simulink model "Edited_MotorXploer"  (R2024b)
settings: Solver=FixedStepAuto  StartTime=0.0  StopTime=10  FixedStep=0.001  RelTol=1e-3
undefined symbols (not defined in the file or in its folder): Blocking, LF, Non
libraries: hdlsllib x5, amg_usbconverter_n_connect_lib x3, dspfdesign x1
settings Model: Creator=beamk  LastModifiedBy=charmil

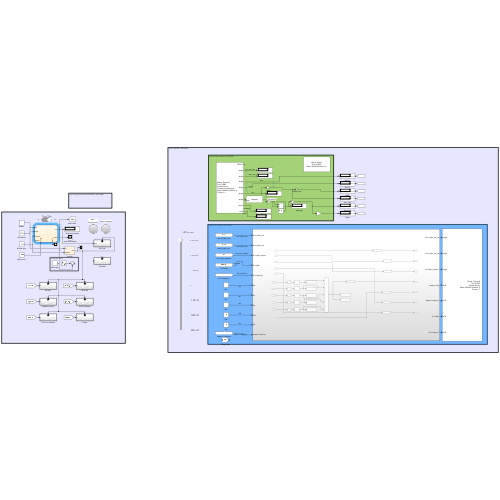
[thumbnail: Simulink's stored preview of the top-level diagram]
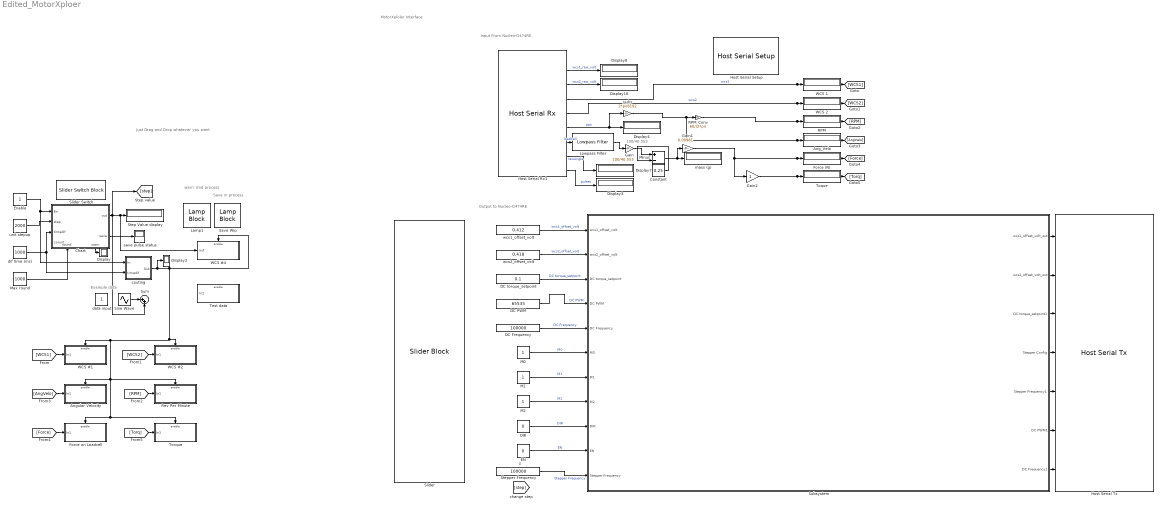
== system Edited_MotorXploer ==
  note: 0
  note: 100/40.553
  note: Just Drag and Drop whatever you want
  note: Output to Nucleo-G474RE
  note: Input From Nucleo-G474RE
  note: MotorXploler Interface
  note: Save in process
  note: Example data
  note: warn:
      | End process
  Ang_Velo : Display
  Angular Velocity : Subsystem  TreatAsAtomicUnit=on
  Chart : Stateflow chart  TreatAsAtomicUnit=on
      settings: PortSchema="{\"entries\":[{\"content\":{\"sides\":[{\"content\":{\"connectorIds\":[\"In2\",\"In3\",\"In4\",\"In5\"]},\"type\":\"ConnectorPlacement.EquallySpacedRectSide\",\"uuid\":\"dac77e3e-29fa-48b2-8dbc-87de7162ff91\"},{\"content\":{\"connectorIds\":[\"Out3\",\"Out2\"],\"side\":\"RIGHT\"},\"type\":\"ConnectorPlacement.EquallySpacedRectSide\",\"uuid\":\"95dcbdb3-8d7f-4284-beec-a5517aef8ac9\"},{\"content\":{\"side\":\"TOP\"},\"type\":\"ConnectorPlacement.EquallySpacedRectSide\",\"uuid\":\"16d4b6a6-1864-4ff8-80c4-a30afaa9113f\"},{\"content\":{\"connectorIds\":[\"In1\",\"Out1\"],\"side\":\"BOTTOM\"},\"type\":\"ConnectorPlacement.EquallySpacedRectSide\",\"uuid\":\"ee49f440-8a25-4cdc-af3c-34657fa2d15f\"}]},\"type\":\"ConnectorPlacement.EquallySpacedConnector\",\"uuid\":\"13973787-06fa-47f1-9425-9f6e417a8e61\"}],\"packageUris\":[\"http://schema.mathworks.com/mf0/Connector/R2020b\"],\"version\":\"1.0\"}"
  Constant : Constant  Value=0.25
  DC Frequency : Constant  Value=100000
  DC PWM : Constant  Value=65535
  DC torque_setpoint : Constant  Value=0.1
  DIR : Constant  Value=0  OutDataTypeStr=uint8
  Display{,2..4,7..8,16} (7 alike) : Display
  EN : Constant  Value=0  OutDataTypeStr=uint8
  Enable : Constant
  Force (N) : Display
  Force on Loadcell : Subsystem  TreatAsAtomicUnit=on
  Gain : Gain  Gain=100/40.553
  Gain1 : Gain  Gain=0.00981
  Gain2 : Gain
  Host Serial Rx1 : amg_usbconverter_n_connect_lib/Host Serial Rx  conf=rx  port=<auto>  baudrate=2000000  databits=8  parity=None  stopbit=1  flowcontrol=None  transfer=Non-Blocking  timeout=5  packetmode=Binary  enableinitialvalues=off  initialvalues=[]  binheader='45'  binterminator='A'  porttype_double=0  porttype_single=6  porttype_int8=0  porttype_uint8=0  porttype_int16=0  porttype_uint16=1  porttype_int32=1  porttype_uint32=0  asciiformat='%f,%f,%d,%d'  rx_asciiterminator="LF (0x0A - \"\\n\")"  tx_asciiterminator="CRLF (0x0D 0x0A - \"\\r\\n\")"  sampletime=-1  enablecustomportlabel=off  cinputportlabel=0  coutputportlabel=A  portpinstr=0  blockid=HostSerialRx1  inputporttype=[]  inputportwidth=[]  inputportlabel={}  outputporttype=[3 1 1 1 1 1 1 5 6]  outputportwidth=[1 1 1 1 1 1 1 1 1]  outputportlabel={'READY','single','single','single','single','single','single','uint16','int32'}  compat=0  optionstring=[]  autoport='COM3'
  Host Serial Setup : amg_usbconverter_n_connect_lib/Host Serial Setup  conf=setup  port=<auto>  baudrate=2000000  databits=8  parity=None  stopbit=1  flowcontrol=None  transfer=Blocking  timeout=2  packetmode=Binary  initialvalues=[]  binheader='7E 7E'  binterminator='03 03'  porttype_double=0  porttype_single=1  porttype_int8=0  porttype_uint8=0  porttype_int16=0  porttype_uint16=0  porttype_int32=0  porttype_uint32=2  asciiformat='%d %u %x'  rx_asciiterminator="CRLF (0x0D 0x0A - \"\\r\\n\")"  tx_asciiterminator="CRLF (0x0D 0x0A - \"\\r\\n\")"  sampletime=-1  enablecustomportlabel=off  cinputportlabel=0  coutputportlabel=A  portpinstr=0  blockid=HostSerialSetup  inputporttype=[]  inputportwidth=[]  inputportlabel={}  outputporttype=[]  outputportwidth=[]  outputportlabel={}  compat=0  optionstring=[]  autoport='COM3'
  Host Serial Tx : amg_usbconverter_n_connect_lib/Host Serial Tx  conf=tx  port=<auto>  baudrate=2000000  databits=8  parity=None  stopbit=1  flowcontrol=None  transfer=Blocking  timeout=2  packetmode=Binary  initialvalues=[]  binheader='45'  binterminator='A'  porttype_double=0  porttype_single=3  porttype_int8=0  porttype_uint8=1  porttype_int16=0  porttype_uint16=0  porttype_int32=3  porttype_uint32=0  asciiformat='%d,%f'  rx_asciiterminator="CRLF (0x0D 0x0A - \"\\r\\n\")"  tx_asciiterminator="CRLF (0x0D 0x0A - \"\\r\\n\")"  sampletime=-1  enablecustomportlabel=off  cinputportlabel=0  coutputportlabel=A  portpinstr=0  blockid=HostSerialTx  inputporttype=[1 1 1 3 6 6 6]  inputportwidth=[1 1 1 1 1 1 1]  inputportlabel={'single','single','single','uint8','int32','int32','int32'}  outputporttype=[]  outputportwidth=[]  outputportlabel={}  compat=0  optionstring=[]  autoport='COM3'
      settings: SourceProductName=aMG USB Converter N
  Lamp1 : LampBlock  LabelPosition=Hide
  Lowpass Filter : dspfdesign/Lowpass Filter  FilterType=FIR  DesignForMinimumOrder=on  FilterOrder=50  PassbandFrequency=0.01  StopbandFrequency=0.1  PassbandRipple=0.1  StopbandAttenuation=80  SampleRateMode=Use normalized frequency (0 to 1)  SampleRate=44100  SimulateUsing=Interpreted execution  roundingMode=Floor  coeffsDataTypeStr=fixdt(1,16)
  M0 : Constant  OutDataTypeStr=uint8
  M1 : Constant
  M2 : Constant  OutDataTypeStr=uint8
  Max round : Constant  Value=1000
  Minus : Sum  Inputs=+-
  RPM : Display
  RPM_Conv : Gain  Gain=60/(2*pi)
  Rev Per Minute : Subsystem  TreatAsAtomicUnit=on
  Save Wip : LampBlock  LabelPosition=Hide
  Sine Wave : Sin  Frequency=20  SampleTime=0
  Slider : SliderBlock  ScaleMin=-65535  ScaleMax=65535
  Slider Switch : SliderSwitchBlock
      settings: Values={{'Off', 'On'}, [0 1]}
  Step Value display : Display
  Stepper Frequency : Constant  Value=100000  VectorParams1D=off
  Subsystem : Subsystem
  Sum : Sum  Inputs=|++
  Test data : Subsystem  TreatAsAtomicUnit=on
  Toque : Display
  Torque : Subsystem  TreatAsAtomicUnit=on
  WCS #1 : Subsystem  TreatAsAtomicUnit=on
  WCS #2 : Subsystem  TreatAsAtomicUnit=on
  WCS #4 : Subsystem  TreatAsAtomicUnit=on
  WCS 1 : Display
  WCS 2 : Display
  couting : Stateflow chart  TreatAsAtomicUnit=on
  data input : Constant
  dif time (ms) : Constant  Value=1000
  mass (g) : Display
  rad/s : Gain  Gain=2*pi/8192
  save pulse status : Display
  unit stepup : Constant  Value=2000
  wcs1_offset_volt : Constant  Value=0.412  OutDataTypeStr=single
  wcs2_offset_volt : Constant  Value=0.418  OutDataTypeStr=single
  wires:
  Host Serial Rx1/2 -> Display8/1  "wcs1_raw_volt"
  Host Serial Rx1/3 -> Display16/1  "wcs2_raw_volt"
  Host Serial Rx1/7 -> Lowpass Filter/1  "loadcell"
  Host Serial Rx1/5 -> [WCS2], WCS 2/1  "wcs2"
  Host Serial Rx1/8 -> Display7/1  "rawAngle"
  rad/s/1 -> [AngVelo], Ang_Velo/1, RPM_Conv/1
  Host Serial Rx1/6 -> Display4/1, rad/s/1  "pps"
  Host Serial Rx1/4 -> [WCS1], WCS 1/1  "wcs1"
  Host Serial Rx1/9 -> Display3/1  "pulses"
  wcs1_offset_volt/1 -> Subsystem/1(wcs1_offset_volt)  "wcs1_offset_volt"
  wcs2_offset_volt/1 -> Subsystem/2(wcs2_offset_volt)  "wcs2_offset_volt"
  DC torque_setpoint/1 -> Subsystem/3(DC torque_setpoint)  "DC torque_setpoint"
  DC PWM/1 -> Subsystem/4(DC PWM)  "DC PWM"
  DC Frequency/1 -> Subsystem/5(DC Frequency)  "DC Frequency"
  M0/1 -> Subsystem/6(M0)  "M0"
  M1/1 -> Subsystem/7(M1)  "M1"
  M2/1 -> Subsystem/8(M2)  "M2"
  DIR/1 -> Subsystem/9(DIR)  "DIR"
  EN/1 -> Subsystem/10(EN)  "EN"
  Subsystem/1(wcs1_offset_volt_out) -> Host Serial Tx/1
  Subsystem/2(wcs2_offset_volt_out) -> Host Serial Tx/2
  Subsystem/3(DC torque_setpoint1) -> Host Serial Tx/3
  Subsystem/4(Stepper Config) -> Host Serial Tx/4
  Subsystem/5(Stepper Frequency1) -> Host Serial Tx/5
  Subsystem/6(DC PWM1) -> Host Serial Tx/6
  Subsystem/7(DC Frequency1) -> Host Serial Tx/7
  Gain/1 -> Minus/1
  Gain1/1 -> Gain2/1, [Force], Force (N)/1
  RPM_Conv/1 -> [RPM], RPM/1
  Sine Wave/1 -> Sum/1
  Chart/2(save) -> save pulse status/1
  dif time (ms)/1 -> couting/2(timedif), Chart/4(timedif)
  Chart/3(out) -> Sum/2, WCS #4/1(out), Step Value display/1, [step]
  Enable/1 -> Chart/2(En), couting/1(In)
  unit stepup/1 -> Chart/3(step)
  Gain2/1 -> [Torq], Toque/1
  [WCS1] -> WCS #1/1(In1)
  [WCS2] -> WCS #2/1(In1)
  [RPM] -> Rev Per Minute/1(In1)
  [Force] -> Force on Loadcell/1(In1)
  [Torq] -> Torque/1(In1)
  Max round/1 -> Chart/1(round)
  Chart/1(warn) -> Display/1
  Lowpass Filter/1 -> Gain/1
  Constant/1 -> Minus/2
  Minus/1 -> Gain1/1, mass (g)/1
  [AngVelo] -> Angular Velocity/1(In1)
  couting/1(Out) -> WCS #4/Enable, WCS #2/Enable, WCS #1/Enable, Angular Velocity/Enable, Rev Per Minute/Enable, Torque/Enable, Force on Loadcell/Enable, Display2/1
  Stepper Frequency/1 -> Subsystem/11(Stepper Frequency)  "Stepper Frequency"

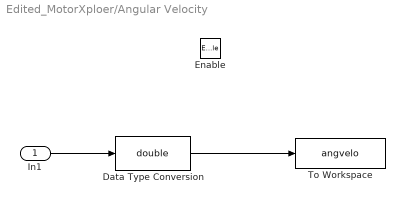
== system Edited_MotorXploer/Angular Velocity ==
  In1 : Inport
  Enable : EnablePort
  Data Type Conversion : DataTypeConversion  OutDataTypeStr=double  SaturateOnIntegerOverflow=off  RndMeth=Floor
  To Workspace : ToWorkspace  VariableName=angvelo  SampleTime=-1
      settings: Save2DSignal=2-D array (concatenate along first dimension)
  wires:
  In1/1 -> Data Type Conversion/1
  Data Type Conversion/1 -> To Workspace/1

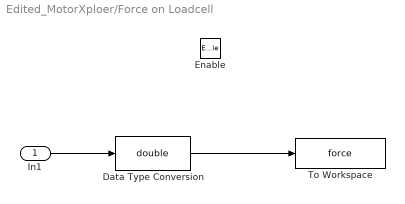
== system Edited_MotorXploer/Force on Loadcell ==
  In1 : Inport
  Enable : EnablePort
  Data Type Conversion : DataTypeConversion  OutDataTypeStr=double  SaturateOnIntegerOverflow=off  RndMeth=Floor
  To Workspace : ToWorkspace  VariableName=force  SampleTime=-1
      settings: Save2DSignal=2-D array (concatenate along first dimension)
  wires:
  In1/1 -> Data Type Conversion/1
  Data Type Conversion/1 -> To Workspace/1

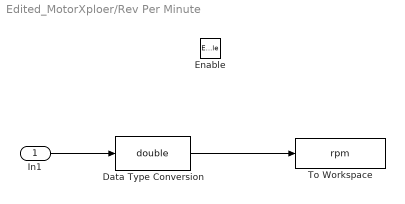
== system Edited_MotorXploer/Rev Per Minute ==
  In1 : Inport
  Enable : EnablePort
  Data Type Conversion : DataTypeConversion  OutDataTypeStr=double  SaturateOnIntegerOverflow=off  RndMeth=Floor
  To Workspace : ToWorkspace  VariableName=rpm  SampleTime=-1
      settings: Save2DSignal=2-D array (concatenate along first dimension)
  wires:
  In1/1 -> Data Type Conversion/1
  Data Type Conversion/1 -> To Workspace/1

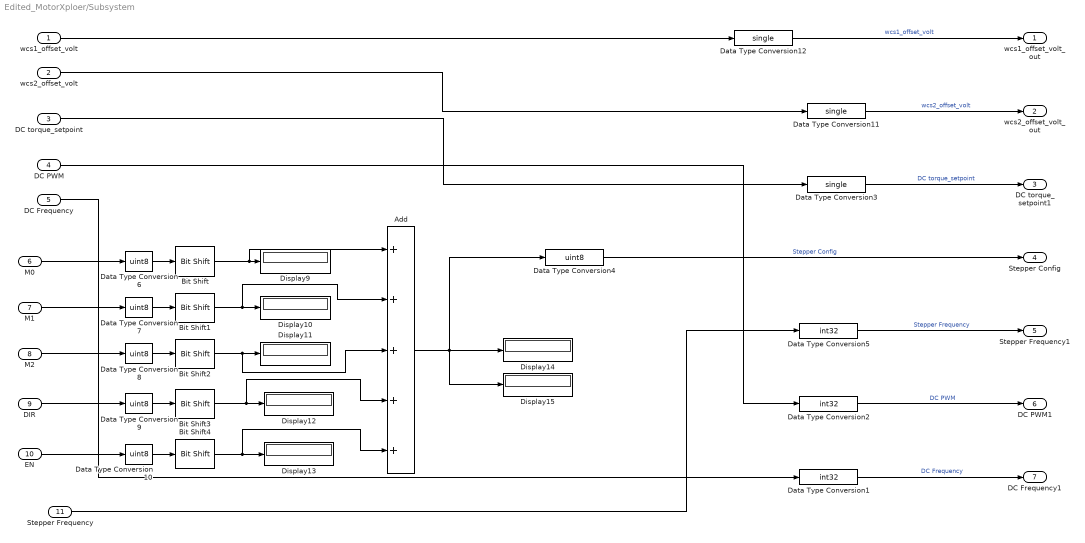
== system Edited_MotorXploer/Subsystem ==
  wcs1_offset_volt : Inport
  wcs2_offset_volt : Inport  Port=2
  DC torque_setpoint : Inport  Port=3
  DC PWM : Inport  Port=4
  DC Frequency : Inport  Port=5
  M0 : Inport  Port=6
  M1 : Inport  Port=7
  M2 : Inport  Port=8
  DIR : Inport  Port=9
  EN : Inport  Port=10
  Stepper Frequency : Inport  Port=11
  Add : Sum  Inputs=+++++
  Bit Shift : hdlsllib/Logic and Bit Operations/Bit Shift  mode=Shift Left Logical  N=4
  Bit Shift1 : hdlsllib/Logic and Bit Operations/Bit Shift  mode=Shift Left Logical  N=3
  Bit Shift2 : hdlsllib/Logic and Bit Operations/Bit Shift  mode=Shift Left Logical  N=2
  Bit Shift3 : hdlsllib/Logic and Bit Operations/Bit Shift  mode=Shift Left Logical  N=1
  Bit Shift4 : hdlsllib/Logic and Bit Operations/Bit Shift  mode=Shift Left Logical  N=0
  Data Type Conversion1 : DataTypeConversion  OutDataTypeStr=int32  SaturateOnIntegerOverflow=off  RndMeth=Floor
  Data Type Conversion{4,6..10} (6 alike) : DataTypeConversion  OutDataTypeStr=uint8  SaturateOnIntegerOverflow=off  RndMeth=Floor
  Data Type Conversion11 : DataTypeConversion  OutDataTypeStr=single  SaturateOnIntegerOverflow=off  RndMeth=Floor
  Data Type Conversion12 : DataTypeConversion  OutDataTypeStr=single  SaturateOnIntegerOverflow=off  RndMeth=Floor
  Data Type Conversion2 : DataTypeConversion  OutDataTypeStr=int32  SaturateOnIntegerOverflow=off  RndMeth=Floor
  Data Type Conversion3 : DataTypeConversion  OutDataTypeStr=single  SaturateOnIntegerOverflow=off  RndMeth=Floor
  Data Type Conversion5 : DataTypeConversion  OutDataTypeStr=int32  SaturateOnIntegerOverflow=off  RndMeth=Floor
  Display{9..15} (7 alike) : Display
      Display10 settings: Format=binary (Stored Integer)
      Display11 settings: Format=binary (Stored Integer)
      Display12 settings: Format=binary (Stored Integer)
      Display13 settings: Format=binary (Stored Integer)
      Display14 settings: Format=binary (Stored Integer)
      Display9 settings: Format=binary (Stored Integer)
  wcs1_offset_volt_out : Outport
  wcs2_offset_volt_out : Outport  Port=2
  DC torque_setpoint1 : Outport  Port=3
  Stepper Config : Outport  Port=4
  Stepper Frequency1 : Outport  Port=5
  DC PWM1 : Outport  Port=6
  DC Frequency1 : Outport  Port=7
  wires:
  Bit Shift/1 -> Display9/1, Add/1
  Data Type Conversion8/1 -> Bit Shift2/1
  EN/1 -> Data Type Conversion10/1
  Data Type Conversion6/1 -> Bit Shift/1
  DC torque_setpoint/1 -> Data Type Conversion3/1
  Data Type Conversion2/1 -> DC PWM1/1  "DC PWM"
  Data Type Conversion7/1 -> Bit Shift1/1
  Data Type Conversion10/1 -> Bit Shift4/1
  DC PWM/1 -> Data Type Conversion2/1
  Bit Shift3/1 -> Display12/1, Add/4
  Data Type Conversion12/1 -> wcs1_offset_volt_out/1  "wcs1_offset_volt"
  Add/1 -> Display15/1, Display14/1, Data Type Conversion4/1
  Bit Shift2/1 -> Display11/1, Add/3
  Stepper Frequency/1 -> Data Type Conversion5/1
  M1/1 -> Data Type Conversion7/1
  Bit Shift1/1 -> Display10/1, Add/2
  Bit Shift4/1 -> Display13/1, Add/5
  M0/1 -> Data Type Conversion6/1
  Data Type Conversion9/1 -> Bit Shift3/1
  Data Type Conversion11/1 -> wcs2_offset_volt_out/1  "wcs2_offset_volt"
  M2/1 -> Data Type Conversion8/1
  wcs1_offset_volt/1 -> Data Type Conversion12/1
  DC Frequency/1 -> Data Type Conversion1/1
  wcs2_offset_volt/1 -> Data Type Conversion11/1
  Data Type Conversion1/1 -> DC Frequency1/1  "DC Frequency"
  DIR/1 -> Data Type Conversion9/1
  Data Type Conversion4/1 -> Stepper Config/1  "Stepper Config"
  Data Type Conversion3/1 -> DC torque_setpoint1/1  "DC torque_setpoint"
  Data Type Conversion5/1 -> Stepper Frequency1/1  "Stepper Frequency"

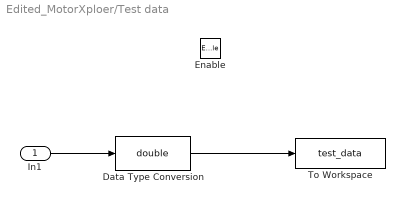
== system Edited_MotorXploer/Test data ==
  In1 : Inport
  Enable : EnablePort
  Data Type Conversion : DataTypeConversion  OutDataTypeStr=double  SaturateOnIntegerOverflow=off  RndMeth=Floor
  To Workspace : ToWorkspace  VariableName=test_data  SampleTime=-1
      settings: Save2DSignal=2-D array (concatenate along first dimension)
  wires:
  In1/1 -> Data Type Conversion/1
  Data Type Conversion/1 -> To Workspace/1

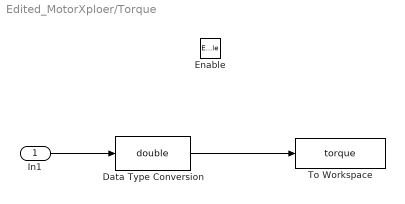
== system Edited_MotorXploer/Torque ==
  In1 : Inport
  Enable : EnablePort
  Data Type Conversion : DataTypeConversion  OutDataTypeStr=double  SaturateOnIntegerOverflow=off  RndMeth=Floor
  To Workspace : ToWorkspace  VariableName=torque  SampleTime=-1
      settings: Save2DSignal=2-D array (concatenate along first dimension)
  wires:
  In1/1 -> Data Type Conversion/1
  Data Type Conversion/1 -> To Workspace/1

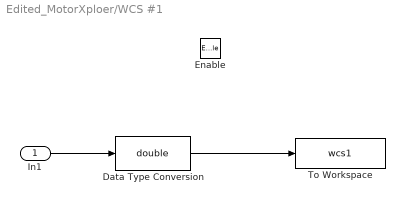
== system Edited_MotorXploer/WCS #1 ==
  In1 : Inport
  Enable : EnablePort
  Data Type Conversion : DataTypeConversion  OutDataTypeStr=double  SaturateOnIntegerOverflow=off  RndMeth=Floor
  To Workspace : ToWorkspace  VariableName=wcs1  SampleTime=-1
      settings: Save2DSignal=2-D array (concatenate along first dimension)
  wires:
  In1/1 -> Data Type Conversion/1
  Data Type Conversion/1 -> To Workspace/1

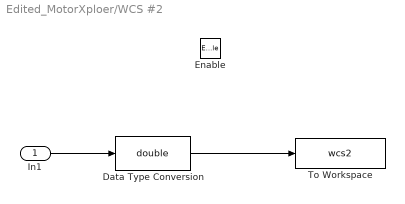
== system Edited_MotorXploer/WCS #2 ==
  In1 : Inport
  Enable : EnablePort
  Data Type Conversion : DataTypeConversion  OutDataTypeStr=double  SaturateOnIntegerOverflow=off  RndMeth=Floor
  To Workspace : ToWorkspace  VariableName=wcs2  SampleTime=-1
      settings: Save2DSignal=2-D array (concatenate along first dimension)
  wires:
  In1/1 -> Data Type Conversion/1
  Data Type Conversion/1 -> To Workspace/1

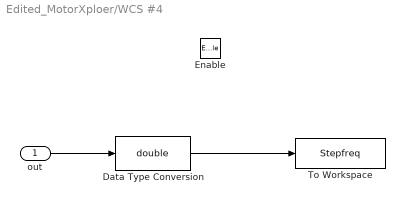
== system Edited_MotorXploer/WCS #4 ==
  out : Inport
  Enable : EnablePort
  Data Type Conversion : DataTypeConversion  OutDataTypeStr=double  SaturateOnIntegerOverflow=off  RndMeth=Floor
  To Workspace : ToWorkspace  VariableName=Stepfreq  SampleTime=-1
      settings: Save2DSignal=2-D array (concatenate along first dimension)
  wires:
  out/1 -> Data Type Conversion/1
  Data Type Conversion/1 -> To Workspace/1

== stateflow chart Edited_MotorXploer/couting ==
  state init
    In;
    Out = 0;
    Count = 1;
    subtime = 0;
    subtime = timedif;
  state Log_dtat
    entry:
    during:
    Count = Count + 1;
    Out = 1;
    exit:
    Out = 0;
  state delay [commented out]
    during:
    subtime = subtime - 1;
  (default) -> init
  Log_dtat -> init : [Count > timedif]
  init -> Log_dtat : [In == 1]
  delay -> Log_dtat [commented out] : [subtime == timedif]
  data: In input; Out output; Count local; timedif input; subtime local

== stateflow chart Edited_MotorXploer/Chart ==
  state warning
    entry:
    warn = 1;
    save = 0;
  state add
    time = 0;
    out = 0;
    couting = 1;
  state oiia
    entry:
    during:
    time = time+1;
    save = 0;
  state addone
    entry:
    out = out + step;
    time = 0;
    save = 1;
    couting = couting + 1;
  state sub
    save = 1;
  state uuu
  oiia -> warning [order 2] : [couting >= round]
  addone -> warning [order 3] : [couting >= round]
  (default) -> add
  addone -> oiia [order 1] : [time == 0]
  oiia -> addone [order 1] : [time > timedif]
  addone -> uuu [order 2] : [En == 0]
  sub -> oiia
  (junction 56) -> addone [order 1] : [time > 0]
  oiia -> uuu [order 3] : [En == 0]
  (junction 56) -> oiia [order 2] : [time == 0]
  add -> sub : [En == 1]
  uuu -> (junction 56) : [En == 1]
  data: warn output; round input; save output; En input; step input; out output; time local; timedif input; corunt input; couting local
